simulink model "Inverse"  (R2013a)
settings: Solver=ode45  StartTime=0.0  StopTime=10.0  RelTol=1e-3
libraries: aerolibutil x2
settings Model: Creator=Rahul Govindaraj  LastModifiedBy=Rahul Govindaraj

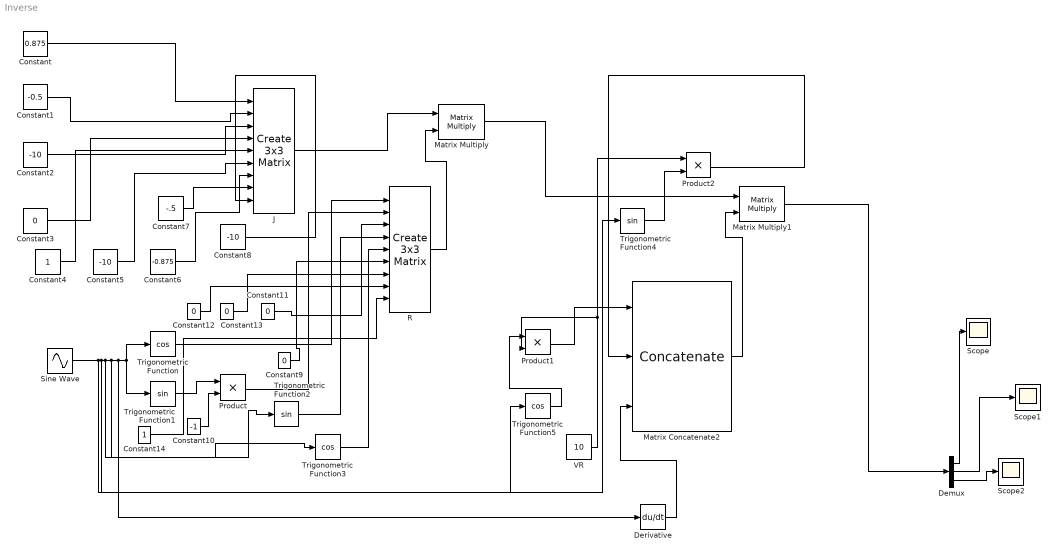
== system Inverse ==
  Constant : Constant  Value=0.875
  Constant1 : Constant  Value=-0.5
  Constant10 : Constant  Value=-1
  Constant{3,9,11..13} (5 alike) : Constant  Value=0
  Constant14 : Constant
  Constant2 : Constant  Value=-10
  Constant4 : Constant
  Constant5 : Constant  Value=-10
  Constant6 : Constant  Value=-0.875
  Constant7 : Constant  Value=-.5
  Constant8 : Constant  Value=-10
  Demux : Demux  Outputs=3
  Derivative : Derivative
  J : aerolibutil/Create 3x3 Matrix
  Matrix Concatenate2 : Concatenate  NumInputs=3  Mode=Multidimensional array
  Matrix Multiply : Product  Multiplication=Matrix(*)
  Matrix Multiply1 : Product  Multiplication=Matrix(*)
  Product : Product
  Product1 : Product
  Product2 : Product
  R : aerolibutil/Create 3x3 Matrix
  Scope : Scope
  Scope1 : Scope
  Scope2 : Scope
      settings: SaveName=ScopeData2
  Sine Wave : Sin  Amplitude=10  SampleTime=0
  Trigonometric Function : Trigonometry  Operator=cos
  Trigonometric Function1 : Trigonometry
  Trigonometric Function2 : Trigonometry
  Trigonometric Function3 : Trigonometry  Operator=cos
  Trigonometric Function4 : Trigonometry
  Trigonometric Function5 : Trigonometry  Operator=cos
  VR : Constant  Value=10
  wires:
  Constant/1 -> J/1
  Constant1/1 -> J/2
  Constant2/1 -> J/3
  Constant3/1 -> J/4
  Constant4/1 -> J/5
  Constant5/1 -> J/6
  Constant6/1 -> J/7
  Constant7/1 -> J/8
  Constant8/1 -> J/9
  Sine Wave/1 -> Trigonometric Function4/1, Trigonometric Function5/1, Trigonometric Function3/1, Trigonometric Function2/1, Derivative/1, Trigonometric Function1/1, Trigonometric Function/1
  Trigonometric Function/1 -> R/1
  Constant10/1 -> Product/2
  Product/1 -> R/2
  Constant11/1 -> R/3
  Constant9/1 -> R/6
  Constant13/1 -> R/7
  Constant12/1 -> R/8
  Constant14/1 -> R/9
  Trigonometric Function5/1 -> Product1/1
  VR/1 -> Product2/1, Product1/2
  Product1/1 -> Matrix Concatenate2/1
  Trigonometric Function4/1 -> Product2/2
  Product2/1 -> Matrix Concatenate2/2
  Derivative/1 -> Matrix Concatenate2/3
  J/1 -> Matrix Multiply/1
  R/1 -> Matrix Multiply/2
  Matrix Concatenate2/1 -> Matrix Multiply1/2
  Matrix Multiply/1 -> Matrix Multiply1/1
  Trigonometric Function1/1 -> Product/1
  Trigonometric Function2/1 -> R/4
  Trigonometric Function3/1 -> R/5
  Matrix Multiply1/1 -> Demux/1
  Demux/1 -> Scope/1
  Demux/2 -> Scope1/1
  Demux/3 -> Scope2/1
